simulink model "MAryAsk"  (Simulink 10.2)
settings: Solver=ode45  StartTime=0.0  StopTime=10.0  RelTol=1e-3  EnableMultiTasking=on
undefined symbols (not defined in the file): fdesignblkfcn, gcbh
libraries: commchan3 x1, commrandsrc2 x1
settings Model: Creator=Abhishek  LastModifiedBy=mluser
settings DataIOCC: LimitDataPoints=on  SignalLoggingSaveFormat=Dataset
settings DebuggingCC: SolverPrmCheckMsg=warning  FcnCallInpInsideContextMsg=error  StateNameClashWarn=warning
settings GRTTargetCC: CombineOutputUpdateFcns=on  GRTInterface=off

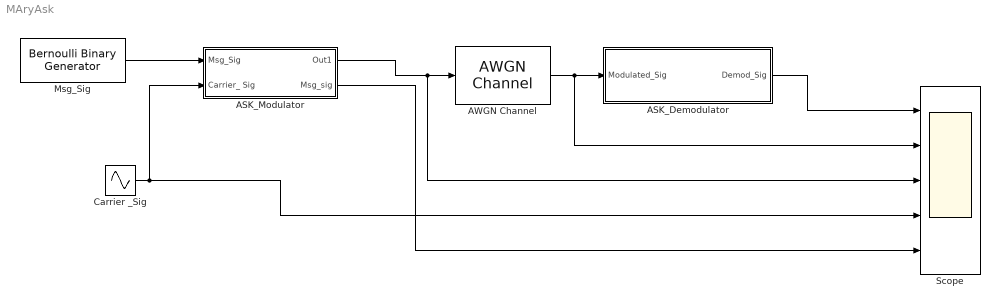
== system MAryAsk ==
  ASK_Demodulator : Subsystem
  ASK_Modulator : Subsystem
  AWGN Channel : commchan3/AWGN Channel  InputProcessing=Columns as channels (frame based)  seed=67  noiseMode="Signal to noise ratio  (Eb/No)"  EbNodB=10  EsNodB=10  SNRdB=10  bitsPerSym=1  Ps=1  Tsym=1  variance=1
  Carrier _Sig : Sin  SineType=Sample based  Amplitude=5  Frequency=100*pi  Samples=50  SampleTime=1/100
  Msg_Sig : commrandsrc2/Bernoulli Binary Generator  P=0.5  seed=61  Ts=1  frameBased=off  sampPerFrame=1  orient=off  outDataType=double  mask(Bernoulli Binary Generator){}
      settings: SourceProductBaseCode=CM
      mask Display:
      | % This is a new mask on top of the base mask.
      | % Use "View base mask" link below to see the base mask.
      | disp('Digital Msg Signal')
  Scope : Scope  NumInputPorts=5
  wires:
  ASK_Modulator/2(Msg_sig) -> Scope/5
  Msg_Sig/1 -> ASK_Modulator/1(Msg_Sig)
  Carrier _Sig/1 -> Scope/4, ASK_Modulator/2(Carrier_ Sig)
  ASK_Demodulator/1(Demod_Sig) -> Scope/1
  AWGN Channel/1 -> Scope/2, ASK_Demodulator/1(Modulated_Sig)
  ASK_Modulator/1(Out1) -> Scope/3, AWGN Channel/1

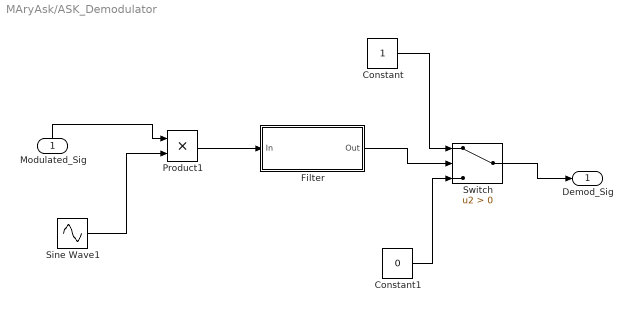
== system MAryAsk/ASK_Demodulator ==
  Modulated_Sig : Inport
  " Filter" : Subsystem  DialogController=fdesignblkfcn  DialogControllerArgs=DataTag1  InitFcn=fdesignblkfcn(gcbh, {'InitFcn'});  mask(Lowpass Filter){}
      mask help: Design a lowpass filter
      settings: CopyFcn=fdesignblkfcn(gcbh, {'CopyFcn'});
      mask Help: helpview(mapfilelocation('dsp'), 'dsplowpassfilter');
      mask Display: disp('Lowpass')
  Constant : Constant
  Constant1 : Constant  Value=0
  Product1 : Product
  Sine Wave1 : Sin  SineType=Sample based  Amplitude=5  Frequency=100*pi  Samples=50  SampleTime=1/100
  Switch : Switch  Criteria=u2 > Threshold
  Demod_Sig : Outport
  wires:
  " Filter"/1(Out) -> Switch/2
  Switch/1 -> Demod_Sig/1
  Sine Wave1/1 -> Product1/2
  Product1/1 -> " Filter"/1(In)
  Constant1/1 -> Switch/3
  Constant/1 -> Switch/1
  Modulated_Sig/1 -> Product1/1

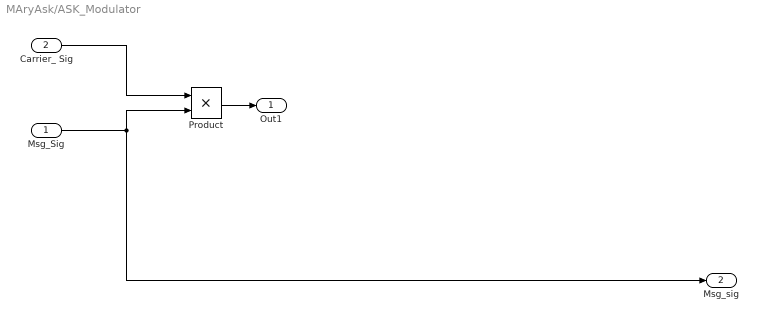
== system MAryAsk/ASK_Modulator ==
  Msg_Sig : Inport
  Carrier_ Sig : Inport  Port=2
  Product : Product
  Out1 : Outport
  Msg_sig : Outport  Port=2
  wires:
  Carrier_ Sig/1 -> Product/1
  Product/1 -> Out1/1
  Msg_Sig/1 -> Product/2, Msg_sig/1

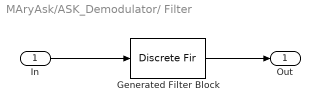
== system MAryAsk/ASK_Demodulator/ Filter ==
  In : Inport
  Generated Filter Block : DiscreteFir  Tag=BlockMethodSubSystem  Coefficients=[0.22210414383484178 0.013518249913456414 0.013700191452328713 0.014207892869318324 0.01421037812449033 0.014545836627592483 0.01421037812449033 0.014207892869318324 0.013700191452328713 0.013518249913456414 0.22210414383484178]
  Out : Outport
  wires:
  In/1 -> Generated Filter Block/1
  Generated Filter Block/1 -> Out/1
